simulink model "Course_autopilot_PIDcontrol"  (R2022a)
settings: Solver=VariableStepAuto  StartTime=0.0  StopTime=10.0  RelTol=1e-3
libraries: mssSimulink x1
settings Model: Creator=XinyiWu  LastModifiedBy=XinyiWu

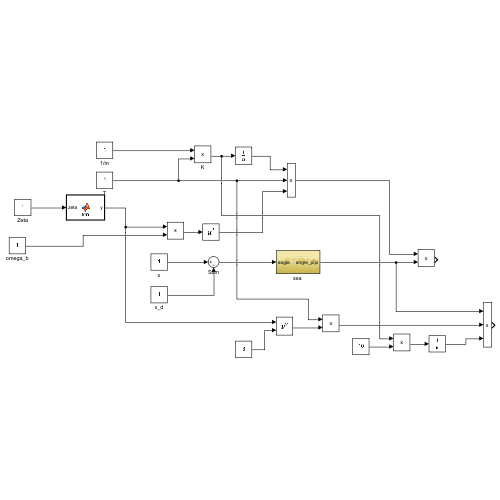
[thumbnail: Simulink's stored preview of the top-level diagram]
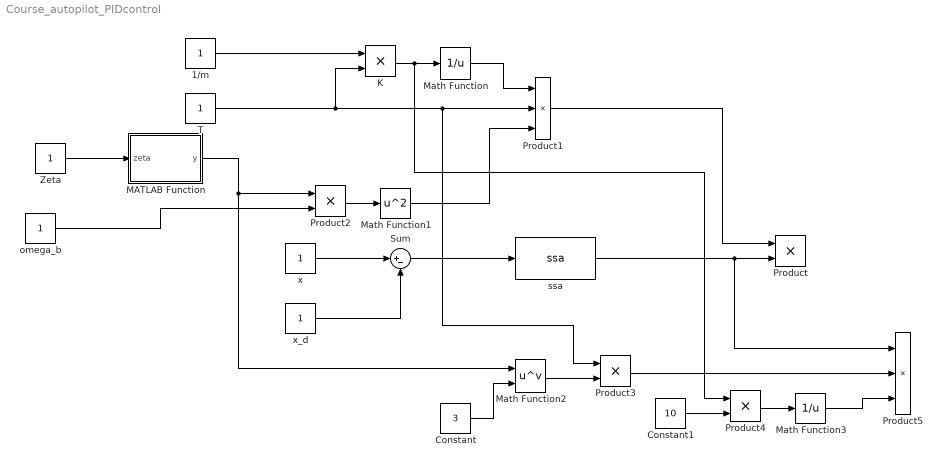
== system Course_autopilot_PIDcontrol ==
  1/m : Constant
  Constant : Constant  Value=3
  Constant1 : Constant  Value=10
  K : Product
  MATLAB Function : MATLAB Function  TreatAsAtomicUnit=on
  Math Function : Math  Operator=reciprocal
  Math Function1 : Math  Operator=square
  Math Function2 : Math  Operator=pow
  Math Function3 : Math  Operator=reciprocal
  Product{,2..4} (4 alike) : Product
  Product1 : Product  Inputs=3
  Product5 : Product  Inputs=3
  Sum : Sum  Inputs=|+-
  T : Constant
  Zeta : Constant
  omega_b : Constant
  "ssa " : mssSimulink/Utilities/Math Operations/ssa  SystemSampleTime=-1  VariantActivationTime=update diagram  Latency=0  AutoFrameSizeCalculation=off
  x : Constant
  x_d : Constant
  wires:
  x/1 -> Sum/1
  Sum/1 -> "ssa "/1
  x_d/1 -> Sum/2
  "ssa "/1 -> Product/2, Product5/1
  1/m/1 -> K/1
  T/1 -> K/2, Product3/1, Product1/2
  K/1 -> Product4/1, Math Function/1
  Math Function/1 -> Product1/1
  MATLAB Function/1(y) -> Product2/1, Math Function2/1
  omega_b/1 -> Product2/2
  Zeta/1 -> MATLAB Function/1(zeta)
  Product2/1 -> Math Function1/1
  Math Function1/1 -> Product1/3
  Product1/1 -> Product/1
  Constant/1 -> Math Function2/2
  Math Function2/1 -> Product3/2
  Constant1/1 -> Product4/2
  Product4/1 -> Math Function3/1
  Math Function3/1 -> Product5/3
  Product3/1 -> Product5/2

== matlab function Course_autopilot_PIDcontrol/MATLAB Function ==
  data: zeta input; y output
function y = fcn(zeta)

y = 1/sqrt(1-2*zeta^2+sqrt(4*zeta^4-4*zeta^2+2));
